simulink library "uavsimBlockset_Cularis_Aerandpropulsion"  (Simulink 8.8)
settings: Solver=ode45  StartTime=0.0  StopTime=10.0  RelTol=1e-3  EnableMultiTasking=on
undefined symbols (not defined in the file): uavsim
libraries: aerolibadyn x1, uavsimBlockset_DerivedAerodynamicConditions x1
settings Model: Creator=mstolle  LastModifiedBy=j.bolting

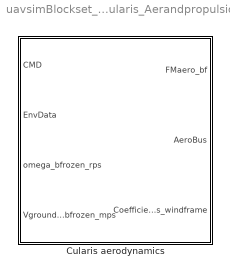
== system uavsimBlockset_Cularis_Aerandpropulsion ==
  Cularis aerodynamics : Subsystem

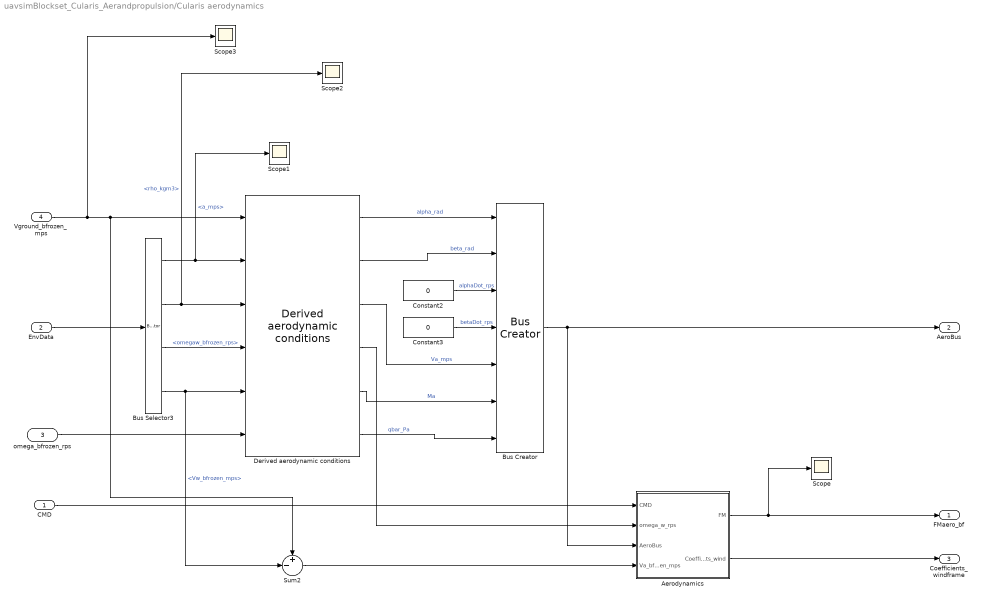
== system uavsimBlockset_Cularis_Aerandpropulsion/Cularis aerodynamics ==
  CMD : Inport  OutDataTypeStr=Bus: CMD
  EnvData : Inport  Port=2  OutDataTypeStr=Bus: Environment
  omega_bfrozen_rps : Inport  Port=3
  Vground_bfrozen_mps : Inport  Port=4
  Aerodynamics : Subsystem
  Bus Selector3 : BusSelector  OutputSignals=a_mps,rho_kgm3,omegaw_bfrozen_rps,Vw_bfrozen_mps
  Bus Creator : BusCreator  Inputs=7
  Constant2 : Constant  Value=0
  Constant3 : Constant  Value=0
  Derived aerodynamic conditions : uavsimBlockset_DerivedAerodynamicConditions/Derived aerodynamic conditions
  Scope{,1..3} (4 alike) : Scope
  Sum2 : Sum  Inputs=+-|  SaturateOnIntegerOverflow=on  InputSameDT=on  OutDataTypeStr=Inherit: Same as first input
  FMaero_bf : Outport
  AeroBus : Outport  Port=2  OutDataTypeStr=Bus: Aero
  Coefficients_windframe : Outport  Port=3
  wires:
  EnvData/1 -> Bus Selector3/1
  omega_bfrozen_rps/1 -> Derived aerodynamic conditions/6
  Aerodynamics/1(FM) -> FMaero_bf/1, Scope/1
  CMD/1 -> Aerodynamics/1(CMD)
  Aerodynamics/2(Coefficients_wind) -> Coefficients_windframe/1
  Bus Selector3/1 -> Derived aerodynamic conditions/2, Scope1/1  "<a_mps>"
  Bus Selector3/2 -> Derived aerodynamic conditions/3, Scope2/1  "<rho_kgm3>"
  Bus Selector3/3 -> Derived aerodynamic conditions/4  "<omegaw_bfrozen_rps>"
  Bus Selector3/4 -> Derived aerodynamic conditions/5, Sum2/2  "<Vw_bfrozen_mps>"
  Constant2/1 -> Bus Creator/3  "alphaDot_rps"
  Constant3/1 -> Bus Creator/4  "betaDot_rps"
  Vground_bfrozen_mps/1 -> Sum2/1, Derived aerodynamic conditions/1, Scope3/1
  Derived aerodynamic conditions/1 -> Bus Creator/1  "alpha_rad"
  Derived aerodynamic conditions/2 -> Bus Creator/2  "beta_rad"
  Derived aerodynamic conditions/3 -> Bus Creator/5  "Va_mps"
  Derived aerodynamic conditions/5 -> Bus Creator/6  "Ma"
  Derived aerodynamic conditions/6 -> Bus Creator/7  "qbar_Pa"
  Bus Creator/1 -> AeroBus/1, Aerodynamics/3(AeroBus)
  Sum2/1 -> Aerodynamics/4(Va_bfrozen_mps)
  Derived aerodynamic conditions/4 -> Aerodynamics/2(omega_w_rps)

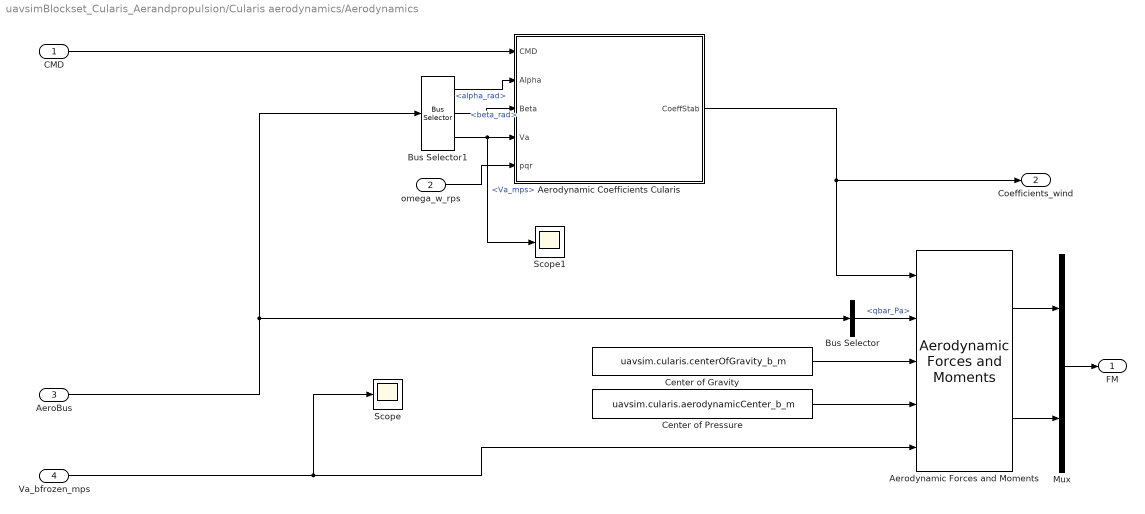
== system uavsimBlockset_Cularis_Aerandpropulsion/Cularis aerodynamics/Aerodynamics ==
  CMD : Inport  OutDataTypeStr=Bus: CMD
  omega_w_rps : Inport  Port=2
  AeroBus : Inport  Port=3  OutDataTypeStr=Bus: Aero
  Va_bfrozen_mps : Inport  Port=4
  Aerodynamic Coefficients Cularis : Subsystem
  "Aerodynamic Forces and Moments " : aerolibadyn/Aerodynamic Forces and Moments   inputAxes=Wind  outputForceAxes=Body  outputMomentAxes=Body  S=uavsim.cularis.S  b=uavsim.cularis.b  cbar=uavsim.cularis.c
  Bus Selector1 : BusSelector  OutputSignals=alpha_rad,beta_rad,Va_mps
  Bus Selector : BusSelector  OutputSignals=qbar_Pa
  Center of Gravity : Constant  Value=uavsim.cularis.centerOfGravity_b_m  SampleTime=0
  Center of Pressure : Constant  Value=uavsim.cularis.aerodynamicCenter_b_m  SampleTime=0
  Mux : Mux  Inputs=2
  Scope : Scope
  Scope1 : Scope
  FM : Outport
  Coefficients_wind : Outport  Port=2
  wires:
  "Aerodynamic Forces and Moments "/2 -> Mux/2
  Aerodynamic Coefficients Cularis/1(CoeffStab) -> "Aerodynamic Forces and Moments "/1, Coefficients_wind/1
  "Aerodynamic Forces and Moments "/1 -> Mux/1
  Center of Gravity/1 -> "Aerodynamic Forces and Moments "/3
  Center of Pressure/1 -> "Aerodynamic Forces and Moments "/4
  CMD/1 -> Aerodynamic Coefficients Cularis/1(CMD)
  Mux/1 -> FM/1
  Bus Selector/1 -> "Aerodynamic Forces and Moments "/2  "<qbar_Pa>"
  AeroBus/1 -> Bus Selector/1, Bus Selector1/1
  Bus Selector1/1 -> Aerodynamic Coefficients Cularis/2(Alpha)  "<alpha_rad>"
  Bus Selector1/2 -> Aerodynamic Coefficients Cularis/3(Beta)  "<beta_rad>"
  Bus Selector1/3 -> Aerodynamic Coefficients Cularis/4(Va), Scope1/1  "<Va_mps>"
  omega_w_rps/1 -> Aerodynamic Coefficients Cularis/5(pqr)
  Va_bfrozen_mps/1 -> Scope/1, "Aerodynamic Forces and Moments "/5

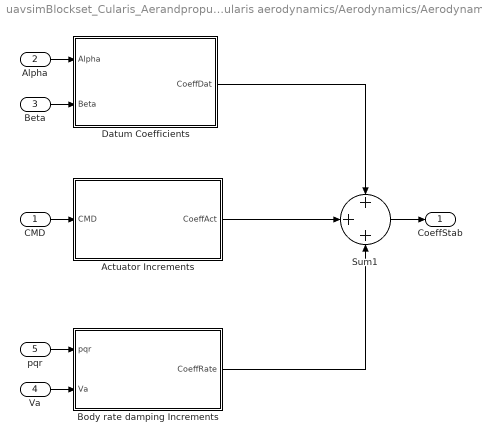
== system uavsimBlockset_Cularis_Aerandpropulsion/Cularis aerodynamics/Aerodynamics/Aerodynamic Coefficients Cularis ==
  CMD : Inport
  Alpha : Inport  Port=2
  Beta : Inport  Port=3
  Va : Inport  Port=4
  pqr : Inport  Port=5
  Actuator Increments : Subsystem
  Body rate damping Increments : Subsystem
  Datum Coefficients : Subsystem
  Sum1 : Sum  Inputs=+++  SaturateOnIntegerOverflow=on  InputSameDT=on  OutDataTypeStr=Inherit: Same as first input
  CoeffStab : Outport
  wires:
  Actuator Increments/1(CoeffAct) -> Sum1/2
  Body rate damping Increments/1(CoeffRate) -> Sum1/3
  Alpha/1 -> Datum Coefficients/1(Alpha)
  Va/1 -> Body rate damping Increments/2(Va)
  pqr/1 -> Body rate damping Increments/1(pqr)
  Beta/1 -> Datum Coefficients/2(Beta)
  CMD/1 -> Actuator Increments/1(CMD)
  Sum1/1 -> CoeffStab/1
  Datum Coefficients/1(CoeffDat) -> Sum1/1

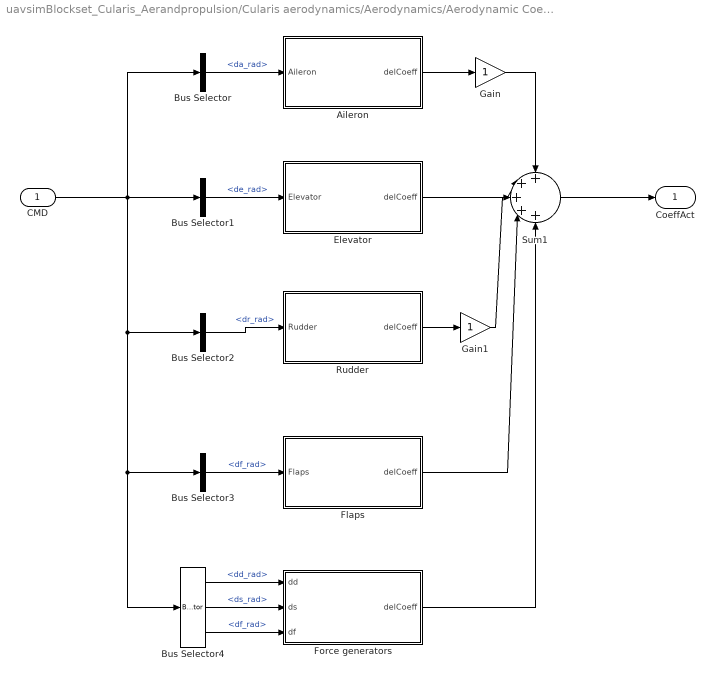
== system uavsimBlockset_Cularis_Aerandpropulsion/Cularis aerodynamics/Aerodynamics/Aerodynamic Coefficients Cularis/Actuator Increments ==
  CMD : Inport
  Aileron : Subsystem
  Bus Selector : BusSelector  OutputSignals=da_rad
  Bus Selector1 : BusSelector  OutputSignals=de_rad
  Bus Selector2 : BusSelector  OutputSignals=dr_rad
  Bus Selector3 : BusSelector  OutputSignals=df_rad
  Bus Selector4 : BusSelector  OutputSignals=dd_rad,ds_rad,df_rad
  Elevator : Subsystem
  Flaps : Subsystem
  Force generators : Subsystem
  Gain : Gain
  Gain1 : Gain
  Rudder : Subsystem
  Sum1 : Sum  Inputs=+++++  SaturateOnIntegerOverflow=on  InputSameDT=on  OutDataTypeStr=Inherit: Same as first input
  CoeffAct : Outport  InitialOutput=0
  wires:
  Force generators/1(delCoeff) -> Sum1/5
  Bus Selector4/3 -> Force generators/3(df)  "<df_rad>"
  Bus Selector4/2 -> Force generators/2(ds)  "<ds_rad>"
  Bus Selector4/1 -> Force generators/1(dd)  "<dd_rad>"
  Flaps/1(delCoeff) -> Sum1/4
  Bus Selector3/1 -> Flaps/1(Flaps)  "<df_rad>"
  Gain1/1 -> Sum1/3
  Gain/1 -> Sum1/1
  Bus Selector/1 -> Aileron/1(Aileron)  "<da_rad>"
  Bus Selector1/1 -> Elevator/1(Elevator)  "<de_rad>"
  Bus Selector2/1 -> Rudder/1(Rudder)  "<dr_rad>"
  CMD/1 -> Bus Selector2/1, Bus Selector3/1, Bus Selector4/1, Bus Selector1/1, Bus Selector/1
  Sum1/1 -> CoeffAct/1
  Rudder/1(delCoeff) -> Gain1/1
  Aileron/1(delCoeff) -> Gain/1
  Elevator/1(delCoeff) -> Sum1/2

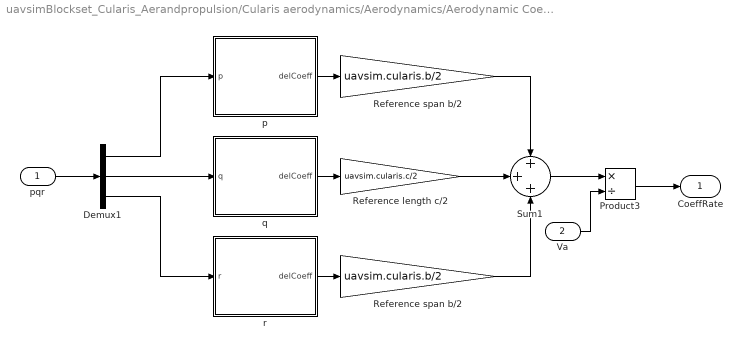
== system uavsimBlockset_Cularis_Aerandpropulsion/Cularis aerodynamics/Aerodynamics/Aerodynamic Coefficients Cularis/Body rate damping Increments ==
  pqr : Inport
  Va : Inport  Port=2
  Demux1 : Demux  Outputs=3
  Product3 : Product  Inputs=*/  SaturateOnIntegerOverflow=on  InputSameDT=on  OutDataTypeStr=Inherit: Same as first input
  Reference length c/2 : Gain  Gain=uavsim.cularis.c/2
  Reference span b/2 : Gain  Gain=uavsim.cularis.b/2
  "Reference span b/2 " : Gain  Gain=uavsim.cularis.b/2
  Sum1 : Sum  Inputs=+++  SaturateOnIntegerOverflow=on  InputSameDT=on  OutDataTypeStr=Inherit: Same as first input
  p : Subsystem
  q : Subsystem
  r : Subsystem
  CoeffRate : Outport  InitialOutput=0
  wires:
  pqr/1 -> Demux1/1
  Demux1/1 -> p/1(p)
  Demux1/2 -> q/1(q)
  Demux1/3 -> r/1(r)
  p/1(delCoeff) -> "Reference span b/2 "/1
  q/1(delCoeff) -> Reference length c/2/1
  r/1(delCoeff) -> Reference span b/2/1
  Product3/1 -> CoeffRate/1
  Sum1/1 -> Product3/1
  Va/1 -> Product3/2
  Reference span b/2/1 -> Sum1/3
  Reference length c/2/1 -> Sum1/2
  "Reference span b/2 "/1 -> Sum1/1

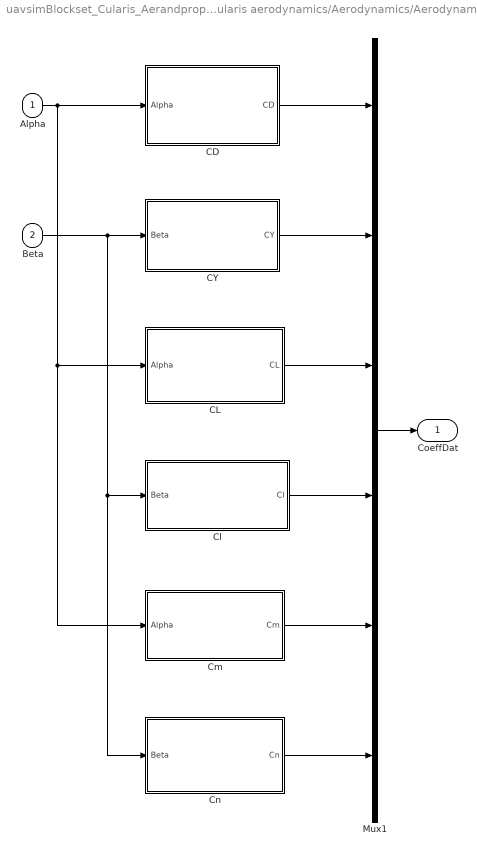
== system uavsimBlockset_Cularis_Aerandpropulsion/Cularis aerodynamics/Aerodynamics/Aerodynamic Coefficients Cularis/Datum Coefficients ==
  Alpha : Inport
  Beta : Inport  Port=2
  CD : Subsystem
  CL : Subsystem
  CY : Subsystem
  Cl : Subsystem
  Cm : Subsystem
  Cn : Subsystem
  Mux1 : Mux  Inputs=6
  CoeffDat : Outport  InitialOutput=0
  wires:
  Alpha/1 -> CD/1(Alpha), CL/1(Alpha), Cm/1(Alpha)
  Mux1/1 -> CoeffDat/1
  Beta/1 -> Cn/1(Beta), Cl/1(Beta), CY/1("Beta ")
  Cn/1(Cn) -> Mux1/6
  Cm/1(Cm) -> Mux1/5
  Cl/1("Cl ") -> Mux1/4
  CY/1(CY) -> Mux1/2
  CD/1(CD) -> Mux1/1
  CL/1(CL) -> Mux1/3

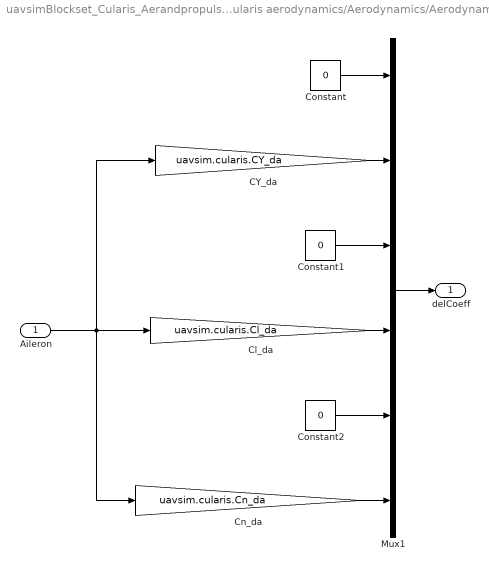
== system uavsimBlockset_Cularis_Aerandpropulsion/Cularis aerodynamics/Aerodynamics/Aerodynamic Coefficients Cularis/Actuator Increments/Aileron ==
  Aileron : Inport
  CY_da : Gain  Gain=uavsim.cularis.CY_da
  Cl_da : Gain  Gain=uavsim.cularis.Cl_da
  Cn_da : Gain  Gain=uavsim.cularis.Cn_da
  Constant : Constant  Value=0
  Constant1 : Constant  Value=0
  Constant2 : Constant  Value=0
  Mux1 : Mux  Inputs=6
  delCoeff : Outport
  wires:
  Constant2/1 -> Mux1/5
  Constant1/1 -> Mux1/3
  Aileron/1 -> Cl_da/1, Cn_da/1, CY_da/1
  Constant/1 -> Mux1/1
  Mux1/1 -> delCoeff/1
  CY_da/1 -> Mux1/2
  Cl_da/1 -> Mux1/4
  Cn_da/1 -> Mux1/6

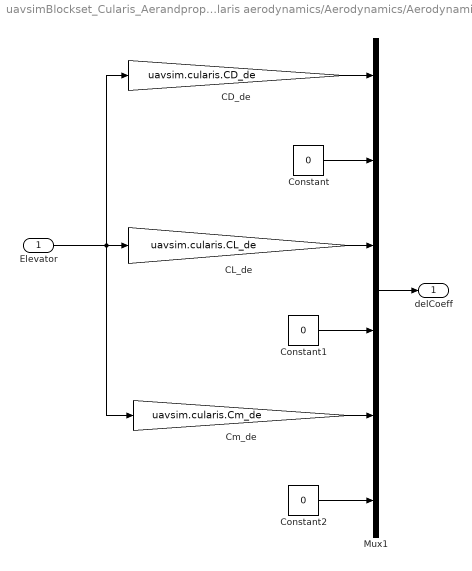
== system uavsimBlockset_Cularis_Aerandpropulsion/Cularis aerodynamics/Aerodynamics/Aerodynamic Coefficients Cularis/Actuator Increments/Elevator ==
  Elevator : Inport
  CD_de : Gain  Gain=uavsim.cularis.CD_de
  CL_de : Gain  Gain=uavsim.cularis.CL_de
  Cm_de : Gain  Gain=uavsim.cularis.Cm_de
  Constant : Constant  Value=0
  Constant1 : Constant  Value=0
  Constant2 : Constant  Value=0
  Mux1 : Mux  Inputs=6
  delCoeff : Outport
  wires:
  Constant2/1 -> Mux1/6
  Constant1/1 -> Mux1/4
  Elevator/1 -> CL_de/1, CD_de/1, Cm_de/1
  CD_de/1 -> Mux1/1
  Mux1/1 -> delCoeff/1
  CL_de/1 -> Mux1/3
  Cm_de/1 -> Mux1/5
  Constant/1 -> Mux1/2

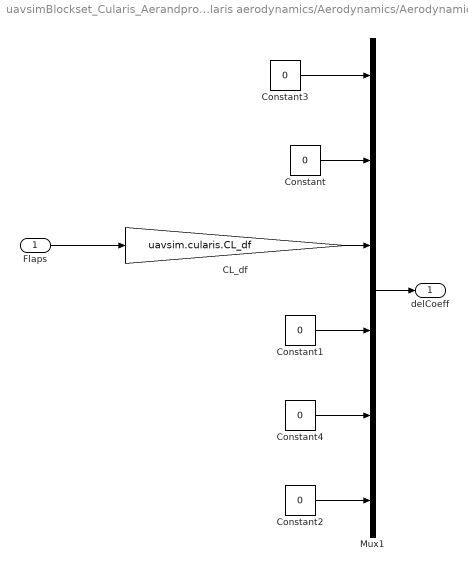
== system uavsimBlockset_Cularis_Aerandpropulsion/Cularis aerodynamics/Aerodynamics/Aerodynamic Coefficients Cularis/Actuator Increments/Flaps ==
  Flaps : Inport
  CL_df : Gain  Gain=uavsim.cularis.CL_df
  Constant{,1..4} (5 alike) : Constant  Value=0
  Mux1 : Mux  Inputs=6
  delCoeff : Outport
  wires:
  Constant4/1 -> Mux1/5
  Constant2/1 -> Mux1/6
  Constant1/1 -> Mux1/4
  Constant3/1 -> Mux1/1
  Mux1/1 -> delCoeff/1
  CL_df/1 -> Mux1/3
  Flaps/1 -> CL_df/1
  Constant/1 -> Mux1/2

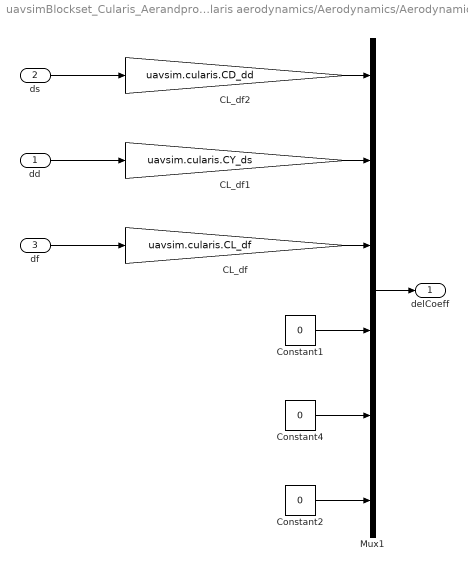
== system uavsimBlockset_Cularis_Aerandpropulsion/Cularis aerodynamics/Aerodynamics/Aerodynamic Coefficients Cularis/Actuator Increments/Force generators ==
  dd : Inport
  ds : Inport  Port=2
  df : Inport  Port=3
  CL_df : Gain  Gain=uavsim.cularis.CL_df
  CL_df1 : Gain  Gain=uavsim.cularis.CY_ds
  CL_df2 : Gain  Gain=uavsim.cularis.CD_dd
  Constant1 : Constant  Value=0
  Constant2 : Constant  Value=0
  Constant4 : Constant  Value=0
  Mux1 : Mux  Inputs=6
  delCoeff : Outport
  wires:
  CL_df1/1 -> Mux1/2
  CL_df2/1 -> Mux1/1
  dd/1 -> CL_df1/1
  df/1 -> CL_df/1
  CL_df/1 -> Mux1/3
  Mux1/1 -> delCoeff/1
  ds/1 -> CL_df2/1
  Constant1/1 -> Mux1/4
  Constant2/1 -> Mux1/6
  Constant4/1 -> Mux1/5

== system uavsimBlockset_Cularis_Aerandpropulsion/Cularis aerodynamics/Aerodynamics/Aerodynamic Coefficients Cularis/Actuator Increments/Rudder ==
  Rudder : Inport
  CY_dr : Gain  Gain=uavsim.cularis.CY_dr
  Cl_dr : Gain  Gain=uavsim.cularis.Cl_dr
  Cn_dr : Gain  Gain=uavsim.cularis.Cn_dr
  Constant : Constant  Value=0
  Constant1 : Constant  Value=0
  Constant2 : Constant  Value=0
  Mux1 : Mux  Inputs=6
  delCoeff : Outport
  wires:
  Constant2/1 -> Mux1/5
  Constant1/1 -> Mux1/3
  Rudder/1 -> Cl_dr/1, Cn_dr/1, CY_dr/1
  Mux1/1 -> delCoeff/1
  CY_dr/1 -> Mux1/2
  Cl_dr/1 -> Mux1/4
  Cn_dr/1 -> Mux1/6
  Constant/1 -> Mux1/1

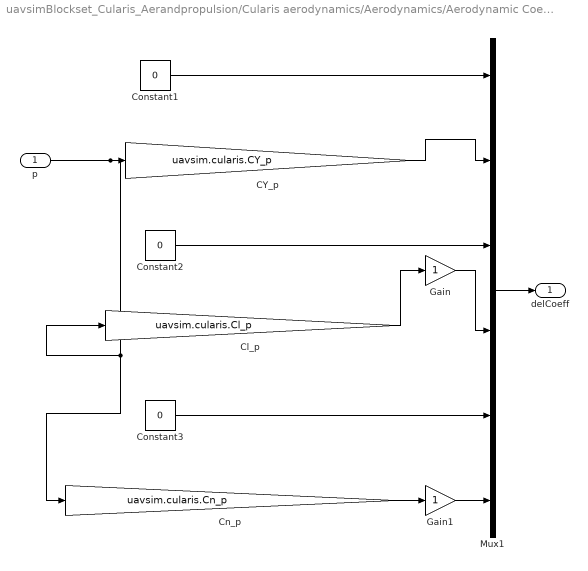
== system uavsimBlockset_Cularis_Aerandpropulsion/Cularis aerodynamics/Aerodynamics/Aerodynamic Coefficients Cularis/Body rate damping Increments/p ==
  p : Inport
  CY_p : Gain  Gain=uavsim.cularis.CY_p
  Cl_p : Gain  Gain=uavsim.cularis.Cl_p
  Cn_p : Gain  Gain=uavsim.cularis.Cn_p
  Constant1 : Constant  Value=0
  Constant2 : Constant  Value=0
  Constant3 : Constant  Value=0
  Gain : Gain
  Gain1 : Gain
  Mux1 : Mux  Inputs=6
  delCoeff : Outport
  wires:
  Gain1/1 -> Mux1/6
  Gain/1 -> Mux1/4
  Constant3/1 -> Mux1/5
  Constant2/1 -> Mux1/3
  Mux1/1 -> delCoeff/1
  Cl_p/1 -> Gain/1
  Cn_p/1 -> Gain1/1
  Constant1/1 -> Mux1/1
  CY_p/1 -> Mux1/2
  p/1 -> CY_p/1, Cl_p/1, Cn_p/1

== system uavsimBlockset_Cularis_Aerandpropulsion/Cularis aerodynamics/Aerodynamics/Aerodynamic Coefficients Cularis/Body rate damping Increments/q ==
  q : Inport
  CD_q : Gain  Gain=uavsim.cularis.CD_q
  CL_q : Gain  Gain=uavsim.cularis.CL_q
  Cm_q : Gain  Gain=uavsim.cularis.Cm_q
  Constant1 : Constant  Value=0
  Constant2 : Constant  Value=0
  Constant3 : Constant  Value=0
  Mux1 : Mux  Inputs=6
  delCoeff : Outport
  wires:
  Constant3/1 -> Mux1/6
  Constant2/1 -> Mux1/4
  Mux1/1 -> delCoeff/1
  q/1 -> CD_q/1, CL_q/1, Cm_q/1
  Constant1/1 -> Mux1/2
  CD_q/1 -> Mux1/1
  CL_q/1 -> Mux1/3
  Cm_q/1 -> Mux1/5

== system uavsimBlockset_Cularis_Aerandpropulsion/Cularis aerodynamics/Aerodynamics/Aerodynamic Coefficients Cularis/Body rate damping Increments/r ==
  r : Inport
  CY_r : Gain  Gain=uavsim.cularis.CY_r
  Cl_r : Gain  Gain=uavsim.cularis.Cl_r
  Cn_r : Gain  Gain=uavsim.cularis.Cn_r
  Constant1 : Constant  Value=0
  Constant2 : Constant  Value=0
  Constant3 : Constant  Value=0
  Mux1 : Mux  Inputs=6
  delCoeff : Outport
  wires:
  Constant3/1 -> Mux1/5
  Constant2/1 -> Mux1/3
  Mux1/1 -> delCoeff/1
  r/1 -> CY_r/1, Cl_r/1, Cn_r/1
  Constant1/1 -> Mux1/1
  CY_r/1 -> Mux1/2
  Cl_r/1 -> Mux1/4
  Cn_r/1 -> Mux1/6

== system uavsimBlockset_Cularis_Aerandpropulsion/Cularis aerodynamics/Aerodynamics/Aerodynamic Coefficients Cularis/Datum Coefficients/CD ==
  Alpha : Inport
  CD_0 : Constant  Value=uavsim.cularis.CD_0
  CL_0 : Constant  Value=uavsim.cularis.CL_0
  CL_alpha : Gain  Gain=uavsim.cularis.CL_alpha
  Product : Product  RndMeth=Zero
  Sum1 : Sum  Inputs=|++
  Sum2 : Sum  Inputs=|++
  sec. order lift contribution : Gain  Gain=1/(pi*uavsim.cularis.oswald*uavsim.cularis.AR )
  CD : Outport
  wires:
  CL_0/1 -> Sum2/1
  Sum2/1 -> Product/2, Product/1
  Product/1 -> sec. order lift contribution/1
  sec. order lift contribution/1 -> Sum1/1
  CD_0/1 -> Sum1/2
  Sum1/1 -> CD/1
  Alpha/1 -> CL_alpha/1
  CL_alpha/1 -> Sum2/2

== system uavsimBlockset_Cularis_Aerandpropulsion/Cularis aerodynamics/Aerodynamics/Aerodynamic Coefficients Cularis/Datum Coefficients/CL ==
  note: CL_0
  Alpha : Inport
  1 : Constant  Value=uavsim.cularis.CL_0
  CL_alpha : Gain  Gain=uavsim.cularis.CL_alpha
  Sum2 : Sum  Inputs=|++
  CL : Outport
  wires:
  Sum2/1 -> CL/1
  1/1 -> Sum2/2
  Alpha/1 -> CL_alpha/1
  CL_alpha/1 -> Sum2/1

== system uavsimBlockset_Cularis_Aerandpropulsion/Cularis aerodynamics/Aerodynamics/Aerodynamic Coefficients Cularis/Datum Coefficients/CY ==
  "Beta " : Inport
  "CY_0 " : Constant  Value=uavsim.cularis.CY_0
  CY_beta : Gain  Gain=uavsim.cularis.CY_beta  SaturateOnIntegerOverflow=on  OutDataTypeStr=Inherit: Same as input  ParamDataTypeStr=Inherit: Same as input
  Sum : Sum  Inputs=|++
  CY : Outport
  wires:
  "Beta "/1 -> CY_beta/1
  Sum/1 -> CY/1
  CY_beta/1 -> Sum/2
  "CY_0 "/1 -> Sum/1

== system uavsimBlockset_Cularis_Aerandpropulsion/Cularis aerodynamics/Aerodynamics/Aerodynamic Coefficients Cularis/Datum Coefficients/Cl ==
  Beta : Inport
  "Cl_0 " : Constant  Value=uavsim.cularis.Cl_0
  Cl_beta : Gain  Gain=uavsim.cularis.Cl_beta  SaturateOnIntegerOverflow=on  OutDataTypeStr=Inherit: Same as input  ParamDataTypeStr=Inherit: Same as input
  Sum1 : Sum  Inputs=|++
  "Cl " : Outport
  wires:
  Cl_beta/1 -> Sum1/1
  "Cl_0 "/1 -> Sum1/2
  Sum1/1 -> "Cl "/1
  Beta/1 -> Cl_beta/1

== system uavsimBlockset_Cularis_Aerandpropulsion/Cularis aerodynamics/Aerodynamics/Aerodynamic Coefficients Cularis/Datum Coefficients/Cm ==
  Alpha : Inport
  Cm_0 : Constant  Value=uavsim.cularis.Cm_0
  Cm_alpha : Gain  Gain=uavsim.cularis.Cm_alpha  SaturateOnIntegerOverflow=on  OutDataTypeStr=Inherit: Same as input  ParamDataTypeStr=Inherit: Same as input
  Sum2 : Sum  Inputs=|++
  Cm : Outport
  wires:
  Cm_0/1 -> Sum2/2
  Sum2/1 -> Cm/1
  Cm_alpha/1 -> Sum2/1
  Alpha/1 -> Cm_alpha/1

== system uavsimBlockset_Cularis_Aerandpropulsion/Cularis aerodynamics/Aerodynamics/Aerodynamic Coefficients Cularis/Datum Coefficients/Cn ==
  Beta : Inport
  Cn_0 : Constant  Value=uavsim.cularis.Cn_0
  Cn_beta : Gain  Gain=uavsim.cularis.Cn_beta  SaturateOnIntegerOverflow=on  OutDataTypeStr=Inherit: Same as input  ParamDataTypeStr=Inherit: Same as input
  Sum3 : Sum  Inputs=|++
  Cn : Outport
  wires:
  Cn_0/1 -> Sum3/2
  Sum3/1 -> Cn/1
  Cn_beta/1 -> Sum3/1
  Beta/1 -> Cn_beta/1
